simulink model "acmotor_vf"  (R2020a)
settings: Solver=ode4  StartTime=0.0  StopTime=4  FixedStep=1e-4  RelTol=1e-3  EnableMultiTasking=on
libraries: powerlib_extras x1
settings Model: Creator=g0305973  LastModifiedBy=TOOLBOX_1
settings DataIOCC: LimitDataPoints=on  SaveFormat=Array  SignalLoggingSaveFormat=ModelDataLogs  ReturnWorkspaceOutputs=off  SignalLoggingName=sigsOut
settings OptimizationCC: ExpressionDepthLimit=2147483647  InitFltsAndDblsToZero=on  LifeSpan=inf
settings DebuggingCC: SaveWithParameterizedLinksMsg=none  UnderspecifiedInitializationDetection=Classic  MergeDetectMultiDrivingBlocksExec=none  SignalResolutionControl=TryResolveAllWithWarning  MultiTaskDSMMsg=warning  MultiTaskCondExecSysMsg=none  FcnCallInpInsideContextMsg=warning  StateNameClashWarn=warning  SFUnexpectedBacktrackingDiag=warning  SFNoUnconditionalDefaultTransitionDiag=warning  SFExecutionAtInitializationDiag=none  ArithmeticOperatorsInVariantConditions=warning
settings HardwareCC: ProdBitPerPointer=32  ProdBitPerSizeT=32  ProdBitPerPtrDiffT=32  ProdLargestAtomicFloat=None  ProdIntDivRoundTo=Undefined  ProdEndianess=Unspecified  ProdWordSize=32  ProdHWDeviceType=32-bit Generic  TargetUnknown=on
settings ModelReferenceCC: PropagateSignalLabelsOutOfModel=off
settings SFSimCC: SimUseLocalCustomCode=off  CustomCodeUndefinedFunction=UseInterfaceOnly
settings RTWCC: RTWUseLocalCustomCode=off
settings CodeAppCC: StateflowObjectComments=on
settings GRTTargetCC: TargetFcnLib=ansi_tfl_tmw.mat  TargetLangStandard=C89/C90 (ANSI)  CombineOutputUpdateFcns=off  GRTInterface=on
settings ConfigComp: CovMetricSettings=dw  CovSaveCumulativeToWorkspaceVar=on  CovSaveSingleToWorkspaceVar=on  CovExternalEMLEnable=off

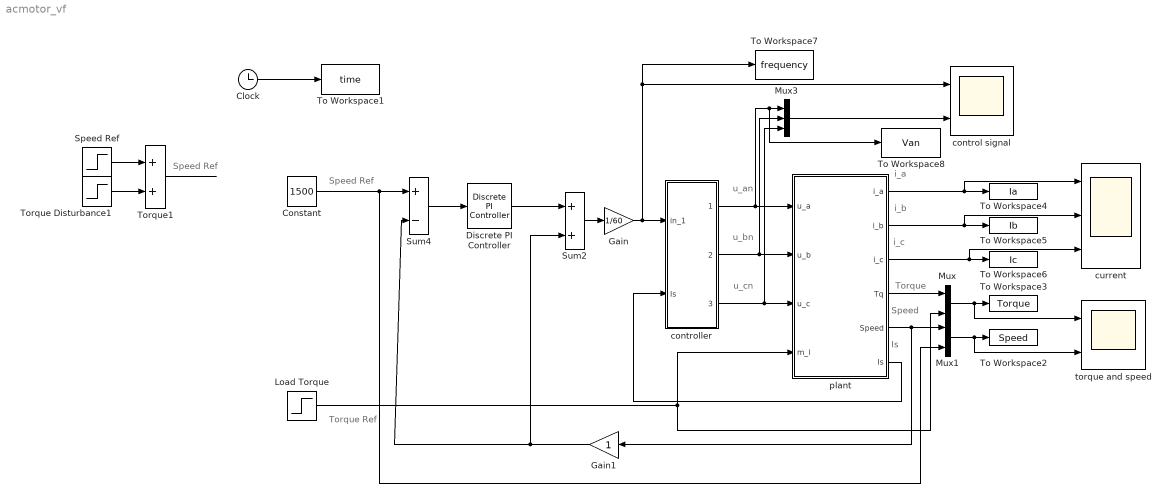
== system acmotor_vf ==
  note: u_cn
  note: u_bn
  note: u_an
  note: Speed
  note: i_b
  note: i_a
  note: i_c
  note: Torque
  note: Speed Ref
  note: Torque Ref
  note: Is
  note: Speed Ref
  Clock : Clock
  Constant : Constant  Value=1500
  Discrete PI Controller : powerlib_extras/Discrete  Control Blocks/Discrete PI Controller  Kp=1  Ki=6  Par_Limits=[2000 0]  Init=0  Ts=100e-6
  Gain : Gain  Gain=1/60
  Gain1 : Gain
  Load Torque : Step  Time=2  After=0
  Mux : Mux  Inputs=2
  Mux1 : Mux  Inputs=2
  Mux3 : Mux  Inputs=3
  Speed Ref : Step  Time=2  Before=1500  After=1200
  Sum2 : Sum  SaturateOnIntegerOverflow=on
  Sum4 : Sum  Inputs=+-  SaturateOnIntegerOverflow=on
  To Workspace1 : ToWorkspace  VariableName=time  SampleTime=1e-4
  To Workspace2 : ToWorkspace  VariableName=Speed  SampleTime=1e-4
  To Workspace3 : ToWorkspace  VariableName=Torque  SampleTime=1e-4
  To Workspace4 : ToWorkspace  VariableName=Ia  SampleTime=1e-4
  To Workspace5 : ToWorkspace  VariableName=Ib  SampleTime=1e-4
  To Workspace6 : ToWorkspace  VariableName=Ic  SampleTime=1e-4
  To Workspace7 : ToWorkspace  VariableName=frequency  SampleTime=1e-4
  To Workspace8 : ToWorkspace  VariableName=Van  SampleTime=1e-4
  Torque Disturbance1 : Step  Time=3  Before=1200  After=900
  Torque1 : Sum  InputSameDT=on  SaturateOnIntegerOverflow=on  OutDataTypeStr=Inherit: Same as first input
  control signal : Scope  NumInputPorts=2
  controller : Subsystem
      mask Display: disp('V/F=c\ncontroller')
  current : Scope  NumInputPorts=3
  plant : Subsystem
      mask init:
      | J = 0.036;
      | B = 0.0015;
      | Ls = 0.4321;	
      | Lh = 0.4125;					
      | Lr = 0.4321;					
      | Rr = 5.6;			
      | Rs = 4.8;			
      | Pp = 2.0;				
      | Tr = Lr / Rr;					
      | Kl = Ls - ((Lh * Lh) / Lr);
      | Kr = Rs + Lh^2 * Rr / Lr^2;
      | 
      | J1 = 0.036;
      | B1 = 0.0015;
      | Ls1 = 0.4321;
      | Lh1 = 0.4125;					
      | Lr1 = 0.4321;		
      | Rr1 = 5.6;					
      | Rs1 = 4.8;					
      | Pp1 = 2.0;					
      | Tr1 = Lr1 / Rr1;			
      | Kl1 = Ls1 - ((Lh1 * Lh1) / Lr1);
      | Kr1 = Rs1 + Lh1^2 * Rr1 / Lr1^2;
      | 
      | INC_LINES = 2048;		
      | FOURFOLD = 4;				
      | SCALE_INC = 2^23;
      | 
      | T_S = 250.0e-6;			
      | SPEED_CTRL_R = 3;	
      | FLUX_CTRL_R = 3;	
      | 
      | US_MAX = 358.0;	
      | ID_MAX = 5.0;		
      | IQ_MAX = 8.0;
      | PSI_REF = 0.93;
      | 
      | a = -B/J;
      | Kt = 3/2*Pp*Lh/Lr*PSI_REF;
      | b = Kt/J;
      | 
      | Kp_i = 15.1;		
      | Tn_i = 0.627;
      | 
      | Kp_n = 0.0312;		
      | Tn_n = 0.0306;
      | 
      | Kp_theta = 75.5;	
      | Tn_theta = 370;
      | 
      | Kp_f = 600.0;		
      | Tn_f = 2.15;
      | 
      | T_speed = 3 * T_S * SPEED_CTRL_R;	
      | 
      | [num_int_speed,den_int_speed] = c2dm([1],[1 0],T_S*SPEED_CTRL_R,'zoh');
      | 
      | [num_int_flux,den_int_flux] = c2dm([1],[1 0],T_S*FLUX_CTRL_R,'zoh');
      | 
      | [num_int_id,den_int_id] = c2dm([1],[1 0],T_S,'zoh');
      | [num_int_iq,den_int_iq] = c2dm([1],[1 0],T_S,'zoh');
      | 
      | [num_fol_flux,den_fol_flux] = c2dm([Lh],[Tr 1],T_S,'zoh');
      | 
      | [num_speed_ref,den_speed_ref] = c2dm([1],[0.036 1],T_S*SPEED_CTRL_R,'zoh');
      | [num_speed,den_speed] = c2dm([1],[T_speed 1],T_S*SPEED_CTRL_R,'zoh');
      | 
      | [num_int_theta,den_int_theta] = c2dm([1],[1 0],T_S,'zoh');
      mask Display: disp('squirrel cage\ninduction motor\nmodel in\nstator frame')
  torque and speed : Scope  NumInputPorts=2
  wires:
  controller/2(out_2) -> plant/2(u_b), Mux3/2
  controller/3(out_3) -> plant/3(u_c), Mux3/3
  plant/1(i_a) -> To Workspace4/1, current/1
  plant/4(Tq) -> Mux/1
  Mux/1 -> To Workspace3/1, torque and speed/1
  plant/3(i_c) -> current/3, To Workspace6/1
  plant/2(i_b) -> To Workspace5/1, current/2
  Clock/1 -> To Workspace1/1
  Load Torque/1 -> Mux/2, plant/4(m_l)
  plant/5(Speed) -> Mux1/1, Gain1/1
  Discrete PI Controller/1 -> Sum2/1
  Sum4/1 -> Discrete PI Controller/1
  Constant/1 -> Sum4/1, Mux1/2
  Mux3/1 -> control signal/2
  Mux1/1 -> To Workspace2/1, torque and speed/2
  Sum2/1 -> Gain/1
  Gain/1 -> controller/1(in_1), control signal/1, To Workspace7/1
  plant/6(Is) -> controller/2(Is)
  Gain1/1 -> Sum4/2, Sum2/2
  controller/1(out_1) -> plant/1(u_a), To Workspace8/1, Mux3/1
  Torque Disturbance1/1 -> Torque1/2
  Speed Ref/1 -> Torque1/1
  Torque1/1 -> ?

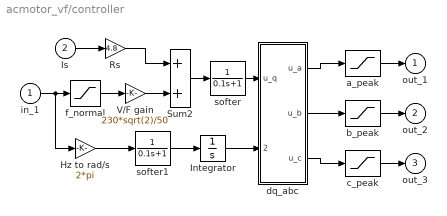
== system acmotor_vf/controller ==
  in_1 : Inport
  Is : Inport  Port=2
  Hz to rad/s : Gain  Gain=2*pi  SaturateOnIntegerOverflow=on  OutDataTypeStr=Inherit: Same as input  ParamDataTypeStr=Inherit: Same as input
  Integrator : Integrator
  Rs : Gain  Gain=4.8  SaturateOnIntegerOverflow=on  OutDataTypeStr=Inherit: Same as input  ParamDataTypeStr=Inherit: Same as input
  Sum2 : Sum  SaturateOnIntegerOverflow=on
  V/F gain : Gain  Gain=230*sqrt(2)/50  SaturateOnIntegerOverflow=on  OutDataTypeStr=Inherit: Same as input  ParamDataTypeStr=Inherit: Same as input
  a_peak : Saturate  UpperLimit=230*sqrt(2)  LowerLimit=-230*sqrt(2)
  b_peak : Saturate  UpperLimit=230*sqrt(2)  LowerLimit=-230*sqrt(2)
  c_peak : Saturate  UpperLimit=230*sqrt(2)  LowerLimit=-230*sqrt(2)
  dq_abc : Subsystem
  f_normal : Saturate  UpperLimit=50  LowerLimit=0
  softer : TransferFcn  Denominator=[0.1 1]
  softer1 : TransferFcn  Denominator=[0.1 1]
  out_1 : Outport  InitialOutput=0
  out_2 : Outport  Port=2  InitialOutput=0
  out_3 : Outport  Port=3  InitialOutput=0
  wires:
  Integrator/1 -> dq_abc/2(eps_fs)
  dq_abc/3(u_c) -> c_peak/1
  dq_abc/2(u_b) -> b_peak/1
  dq_abc/1(u_a) -> a_peak/1
  a_peak/1 -> out_1/1
  b_peak/1 -> out_2/1
  c_peak/1 -> out_3/1
  Hz to rad/s/1 -> softer1/1
  f_normal/1 -> V/F gain/1
  in_1/1 -> Hz to rad/s/1, f_normal/1
  softer/1 -> dq_abc/1(u_q)
  softer1/1 -> Integrator/1
  Sum2/1 -> softer/1
  V/F gain/1 -> Sum2/2
  Is/1 -> Rs/1
  Rs/1 -> Sum2/1

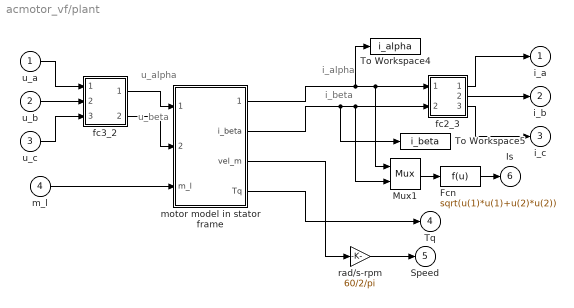
== system acmotor_vf/plant ==
  note: u_beta
  note: u_alpha
  note: i_alpha
  note: i_beta
  u_a : Inport
  u_b : Inport  Port=2
  u_c : Inport  Port=3
  m_l : Inport  Port=4
  Fcn : Fcn  Expr=sqrt(u(1)*u(1)+u(2)*u(2))
  Mux1 : Mux  Inputs=2
  To Workspace4 : ToWorkspace  VariableName=i_alpha
      settings: MaxDataPoints=20000
  To Workspace5 : ToWorkspace  VariableName=i_beta
      settings: MaxDataPoints=20000
  "fc2_3 " : Subsystem
  "fc3_2 " : Subsystem
  motor model in stator frame : Subsystem
  rad/s-rpm : Gain  Gain=60/2/pi  SaturateOnIntegerOverflow=on  OutDataTypeStr=Inherit: Same as input  ParamDataTypeStr=Inherit: Same as input
  i_a : Outport
  i_b : Outport  Port=2
  i_c : Outport  Port=3
  Tq : Outport  Port=4
  Speed : Outport  Port=5
  Is : Outport  Port=6
  wires:
  m_l/1 -> motor model in stator frame/3(m_l)
  "fc3_2 "/1("u_alpha ") -> motor model in stator frame/1(u_alpha)
  "fc3_2 "/2("u_beta ") -> motor model in stator frame/2(u_beta)
  motor model in stator frame/3(vel_m) -> rad/s-rpm/1
  motor model in stator frame/4(Tq) -> Tq/1
  rad/s-rpm/1 -> Speed/1
  u_b/1 -> "fc3_2 "/2(u_b)
  u_a/1 -> "fc3_2 "/1(u_a)
  u_c/1 -> "fc3_2 "/3(u_c)
  "fc2_3 "/1("i_a ") -> i_a/1
  "fc2_3 "/2("i_b ") -> i_b/1
  "fc2_3 "/3("i_c ") -> i_c/1
  motor model in stator frame/1("i_alpha ") -> To Workspace4/1, "fc2_3 "/1(i_alpha), Mux1/1
  motor model in stator frame/2("i_beta ") -> To Workspace5/1, "fc2_3 "/2(i_beta), Mux1/2
  Mux1/1 -> Fcn/1
  Fcn/1 -> Is/1

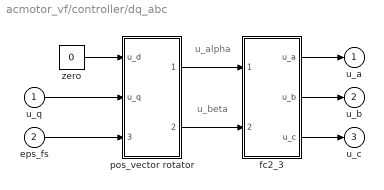
== system acmotor_vf/controller/dq_abc ==
  note: u_alpha
  note: u_beta
  u_q : Inport
  eps_fs : Inport  Port=2
  fc2_3 : Subsystem
  pos_vector rotator : Subsystem
  "zero  " : Constant  Value=0
  u_a : Outport  InitialOutput=0
  u_b : Outport  Port=2  InitialOutput=0
  u_c : Outport  Port=3  InitialOutput=0
  wires:
  pos_vector rotator/1("u_alpha ") -> fc2_3/1(u_alpha)
  pos_vector rotator/2("u_beta ") -> fc2_3/2(u_beta)
  u_q/1 -> pos_vector rotator/2(u_q)
  eps_fs/1 -> pos_vector rotator/3(eps_fs)
  fc2_3/1("u_a ") -> u_a/1
  fc2_3/2("u_b ") -> u_b/1
  fc2_3/3("u_c ") -> u_c/1
  "zero  "/1 -> pos_vector rotator/1(u_d)

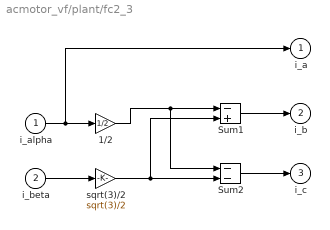
== system acmotor_vf/plant/fc2_3  ==
  i_alpha : Inport
  i_beta : Inport  Port=2
  1/2 : Gain  Gain=1/2  SaturateOnIntegerOverflow=on  OutDataTypeStr=Inherit: Same as input  ParamDataTypeStr=Inherit: Same as input
  Sum1 : Sum  Inputs=-+  InputSameDT=on  SaturateOnIntegerOverflow=on  OutDataTypeStr=Inherit: Same as first input
  Sum2 : Sum  Inputs=--  InputSameDT=on  SaturateOnIntegerOverflow=on  OutDataTypeStr=Inherit: Same as first input
  sqrt(3)/2 : Gain  Gain=sqrt(3)/2  SaturateOnIntegerOverflow=on  OutDataTypeStr=Inherit: Same as input  ParamDataTypeStr=Inherit: Same as input
  "i_a " : Outport
  "i_b " : Outport  Port=2
  "i_c " : Outport  Port=3
  wires:
  sqrt(3)/2/1 -> Sum1/2, Sum2/2
  1/2/1 -> Sum1/1, Sum2/1
  Sum2/1 -> "i_c "/1
  Sum1/1 -> "i_b "/1
  i_alpha/1 -> 1/2/1, "i_a "/1
  i_beta/1 -> sqrt(3)/2/1

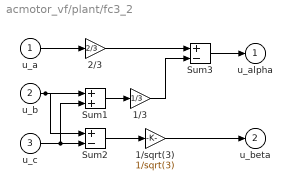
== system acmotor_vf/plant/fc3_2  ==
  u_a : Inport
  u_b : Inport  Port=2
  u_c : Inport  Port=3
  1/3 : Gain  Gain=1/3  SaturateOnIntegerOverflow=on  OutDataTypeStr=Inherit: Same as input  ParamDataTypeStr=Inherit: Same as input
  1/sqrt(3) : Gain  Gain=1/sqrt(3)  SaturateOnIntegerOverflow=on  OutDataTypeStr=Inherit: Same as input  ParamDataTypeStr=Inherit: Same as input
  2/3 : Gain  Gain=2/3  SaturateOnIntegerOverflow=on  OutDataTypeStr=Inherit: Same as input  ParamDataTypeStr=Inherit: Same as input
  Sum1 : Sum  InputSameDT=on  SaturateOnIntegerOverflow=on  OutDataTypeStr=Inherit: Same as first input
  Sum2 : Sum  Inputs=+-  InputSameDT=on  SaturateOnIntegerOverflow=on  OutDataTypeStr=Inherit: Same as first input
  Sum3 : Sum  Inputs=+-  InputSameDT=on  SaturateOnIntegerOverflow=on  OutDataTypeStr=Inherit: Same as first input
  "u_alpha " : Outport
  "u_beta " : Outport  Port=2
  wires:
  Sum1/1 -> 1/3/1
  1/3/1 -> Sum3/2
  u_a/1 -> 2/3/1
  2/3/1 -> Sum3/1
  Sum3/1 -> "u_alpha "/1
  u_b/1 -> Sum1/1, Sum2/1
  u_c/1 -> Sum1/2, Sum2/2
  Sum2/1 -> 1/sqrt(3)/1
  1/sqrt(3)/1 -> "u_beta "/1

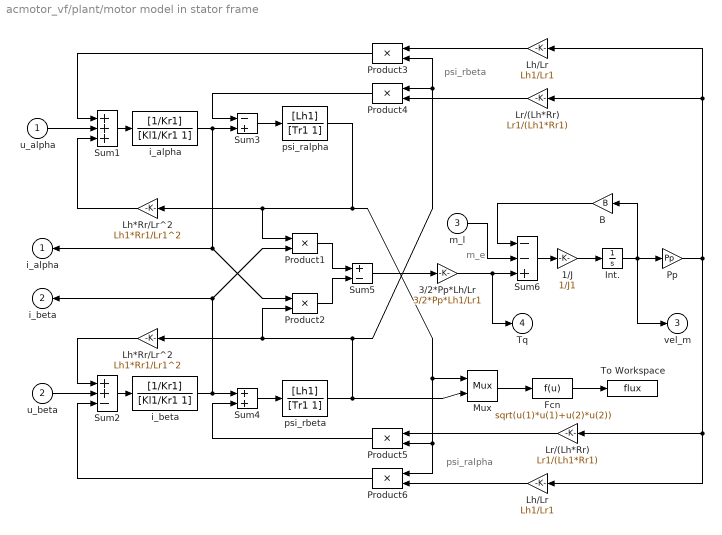
== system acmotor_vf/plant/motor model in stator frame ==
  note: psi_ralpha
  note: psi_rbeta
  note: m_e
  u_alpha : Inport
  u_beta : Inport  Port=2
  m_l : Inport  Port=3
  1/J : Gain  Gain=1/J1  SaturateOnIntegerOverflow=on  OutDataTypeStr=Inherit: Same as input  ParamDataTypeStr=Inherit: Same as input
  3/2*Pp*Lh/Lr : Gain  Gain=3/2*Pp*Lh1/Lr1  SaturateOnIntegerOverflow=on  OutDataTypeStr=Inherit: Same as input  ParamDataTypeStr=Inherit: Same as input
  B : Gain  Gain=B  SaturateOnIntegerOverflow=on  OutDataTypeStr=Inherit: Same as input  ParamDataTypeStr=Inherit: Same as input
  Fcn : Fcn  Expr=sqrt(u(1)*u(1)+u(2)*u(2))
  Int. : Integrator
  Lh*Rr/Lr^2 : Gain  Gain=Lh1*Rr1/Lr1^2  SaturateOnIntegerOverflow=on  OutDataTypeStr=Inherit: Same as input  ParamDataTypeStr=Inherit: Same as input
  "Lh*Rr/Lr^2 " : Gain  Gain=Lh1*Rr1/Lr1^2  SaturateOnIntegerOverflow=on  OutDataTypeStr=Inherit: Same as input  ParamDataTypeStr=Inherit: Same as input
  Lh/Lr : Gain  Gain=Lh1/Lr1  SaturateOnIntegerOverflow=on  OutDataTypeStr=Inherit: Same as input  ParamDataTypeStr=Inherit: Same as input
  "Lh/Lr " : Gain  Gain=Lh1/Lr1  SaturateOnIntegerOverflow=on  OutDataTypeStr=Inherit: Same as input  ParamDataTypeStr=Inherit: Same as input
  Lr/(Lh*Rr) : Gain  Gain=Lr1/(Lh1*Rr1)  SaturateOnIntegerOverflow=on  OutDataTypeStr=Inherit: Same as input  ParamDataTypeStr=Inherit: Same as input
  "Lr/(Lh*Rr) " : Gain  Gain=Lr1/(Lh1*Rr1)  SaturateOnIntegerOverflow=on  OutDataTypeStr=Inherit: Same as input  ParamDataTypeStr=Inherit: Same as input
  Mux : Mux  Inputs=2
  Pp : Gain  Gain=Pp  SaturateOnIntegerOverflow=on  OutDataTypeStr=Inherit: Same as input  ParamDataTypeStr=Inherit: Same as input
  Product{1..6} (6 alike) : Product  InputSameDT=on  SaturateOnIntegerOverflow=on  OutDataTypeStr=Inherit: Same as first input
  Sum1 : Sum  Inputs=+++  InputSameDT=on  SaturateOnIntegerOverflow=on  OutDataTypeStr=Inherit: Same as first input
  Sum2 : Sum  Inputs=++-  InputSameDT=on  SaturateOnIntegerOverflow=on  OutDataTypeStr=Inherit: Same as first input
  Sum3 : Sum  Inputs=-+  InputSameDT=on  SaturateOnIntegerOverflow=on  OutDataTypeStr=Inherit: Same as first input
  Sum4 : Sum  InputSameDT=on  SaturateOnIntegerOverflow=on  OutDataTypeStr=Inherit: Same as first input
  Sum5 : Sum  Inputs=+-  InputSameDT=on  SaturateOnIntegerOverflow=on  OutDataTypeStr=Inherit: Same as first input
  Sum6 : Sum  Inputs=--+  InputSameDT=on  SaturateOnIntegerOverflow=on  OutDataTypeStr=Inherit: Same as first input
  To Workspace : ToWorkspace  VariableName=flux  SampleTime=1e-4
  i_alpha : TransferFcn  Numerator=[1/Kr1]  Denominator=[Kl1/Kr1 1]
  i_beta : TransferFcn  Numerator=[1/Kr1]  Denominator=[Kl1/Kr1 1]
  psi_ralpha : TransferFcn  Numerator=[Lh1]  Denominator=[Tr1 1]
  psi_rbeta : TransferFcn  Numerator=[Lh1]  Denominator=[Tr1 1]
  "i_alpha " : Outport
  "i_beta " : Outport  Port=2
  vel_m : Outport  Port=3
  Tq : Outport  Port=4
  wires:
  Sum6/1 -> 1/J/1
  1/J/1 -> Int./1
  Product4/1 -> Sum3/1
  Lr/(Lh*Rr)/1 -> Product4/2
  Product5/1 -> Sum4/2
  "Lh/Lr "/1 -> Product6/2
  Product6/1 -> Sum2/3
  Product3/1 -> Sum1/1
  "Lr/(Lh*Rr) "/1 -> Product5/1
  Lh/Lr/1 -> Product3/1
  Sum5/1 -> 3/2*Pp*Lh/Lr/1
  Sum4/1 -> psi_rbeta/1
  Sum3/1 -> psi_ralpha/1
  "Lh*Rr/Lr^2 "/1 -> Sum2/1
  Lh*Rr/Lr^2/1 -> Sum1/3
  Sum2/1 -> i_beta/1
  Sum1/1 -> i_alpha/1
  u_beta/1 -> Sum2/2
  u_alpha/1 -> Sum1/2
  i_beta/1 -> Sum4/1, Product1/2, "i_beta "/1
  Product1/1 -> Sum5/1
  Product2/1 -> Sum5/2
  i_alpha/1 -> Sum3/2, Product2/1, "i_alpha "/1
  psi_ralpha/1 -> Lh*Rr/Lr^2/1, Product1/1, Product6/1, Product5/2, Mux/1
  Int./1 -> Pp/1, vel_m/1, B/1
  3/2*Pp*Lh/Lr/1 -> Tq/1, Sum6/3
  Pp/1 -> "Lh/Lr "/1, "Lr/(Lh*Rr) "/1, Lh/Lr/1, Lr/(Lh*Rr)/1
  m_l/1 -> Sum6/2
  B/1 -> Sum6/1
  Mux/1 -> Fcn/1
  Fcn/1 -> To Workspace/1
  psi_rbeta/1 -> Product3/2, Product4/1, "Lh*Rr/Lr^2 "/1, Product2/2, Mux/2

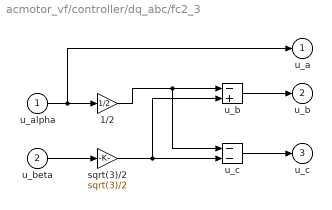
== system acmotor_vf/controller/dq_abc/fc2_3 ==
  u_alpha : Inport
  u_beta : Inport  Port=2
  1/2 : Gain  Gain=1/2  SaturateOnIntegerOverflow=on  OutDataTypeStr=Inherit: Same as input  ParamDataTypeStr=Inherit: Same as input
  sqrt(3)/2 : Gain  Gain=sqrt(3)/2  SaturateOnIntegerOverflow=on  OutDataTypeStr=Inherit: Same as input  ParamDataTypeStr=Inherit: Same as input
  u_b : Sum  Inputs=-+  InputSameDT=on  SaturateOnIntegerOverflow=on  OutDataTypeStr=Inherit: Same as first input
  u_c : Sum  Inputs=--  InputSameDT=on  SaturateOnIntegerOverflow=on  OutDataTypeStr=Inherit: Same as first input
  "u_a " : Outport  InitialOutput=0
  "u_b " : Outport  Port=2  InitialOutput=0
  "u_c " : Outport  Port=3  InitialOutput=0
  wires:
  u_c/1 -> "u_c "/1
  u_b/1 -> "u_b "/1
  1/2/1 -> u_b/1, u_c/1
  sqrt(3)/2/1 -> u_b/2, u_c/2
  u_beta/1 -> sqrt(3)/2/1
  u_alpha/1 -> 1/2/1, "u_a "/1

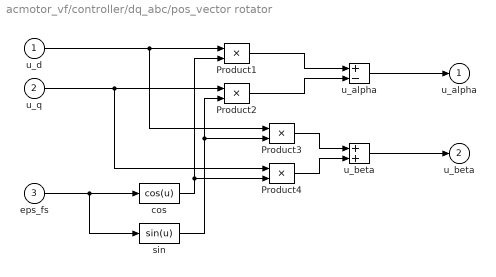
== system acmotor_vf/controller/dq_abc/pos_vector rotator ==
  u_d : Inport
  u_q : Inport  Port=2
  eps_fs : Inport  Port=3
  Product{1..4} (4 alike) : Product  InputSameDT=on  SaturateOnIntegerOverflow=on  OutDataTypeStr=Inherit: Same as first input
  cos : Fcn  Expr=cos(u)
  sin : Fcn  Expr=sin(u)
  u_alpha : Sum  Inputs=+-  InputSameDT=on  SaturateOnIntegerOverflow=on  OutDataTypeStr=Inherit: Same as first input
  u_beta : Sum  InputSameDT=on  SaturateOnIntegerOverflow=on  OutDataTypeStr=Inherit: Same as first input
  "u_alpha " : Outport  InitialOutput=0
  "u_beta " : Outport  Port=2  InitialOutput=0
  wires:
  u_alpha/1 -> "u_alpha "/1
  u_beta/1 -> "u_beta "/1
  eps_fs/1 -> cos/1, sin/1
  Product4/1 -> u_beta/2
  Product3/1 -> u_beta/1
  u_q/1 -> Product2/1, Product4/1
  u_d/1 -> Product1/1, Product3/1
  Product2/1 -> u_alpha/2
  Product1/1 -> u_alpha/1
  sin/1 -> Product2/2, Product3/2
  cos/1 -> Product1/2, Product4/2
